simulink library "lib_finite_difference_filtered_derivative"  (R2023a)
settings: Solver=VariableStepAuto  StartTime=0.0  StopTime=10.0  RelTol=1e-3
undefined symbols (not defined in the file): bit
libraries: lib_conversion x4, lib_finite_difference_derivative x1, lib_iir_filter x1
settings Model: Creator=RAN2OFO  LastModifiedBy=xiaoqiang.yuan
settings OptimizationCC: ReuseModelBlockBuffer=off

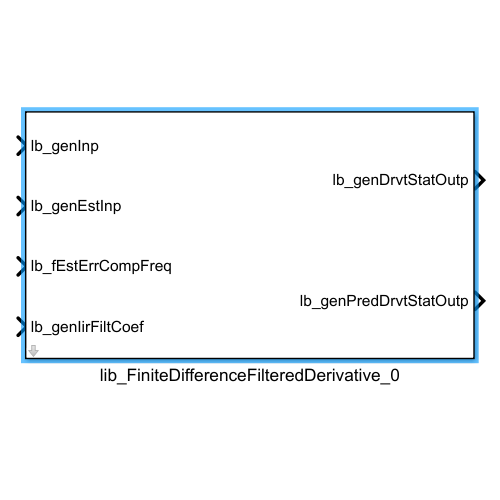
[thumbnail: Simulink's stored preview of the top-level diagram]
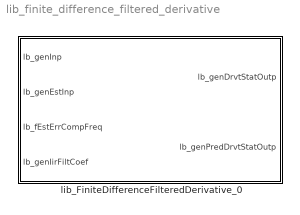
== system lib_finite_difference_filtered_derivative ==
  lib_FiniteDifferenceFilteredDerivative_0 : Subsystem  mask{lb_parSampTime=0.0005, lb_parInpMaxVal=100, lb_parInpEstErrMaxVal=0.1, lb_parInpDiffMaxVal=0.1, lb_parMaxEstErrCompFreq=4000, lb_parFltrCoefMaxVal=0.7, lb_genOutpUpLim=5000, lb_genOutpLowLim=-5000, lb_parOutpPekPhy=4096, lb_parAngInpMode=on, lb_parOutpDataType=fixdt(1,16,2^-3,0)}
      mask prompts: lb_parSampTime "Sampling time [s]:"; lb_parInpMaxVal "Maximum input [iu]:"; lb_parInpEstErrMaxVal "Maximum input estimation error [iu]:"; lb_parInpDiffMaxVal "Maximum input variation [iu]:"; lb_parMaxEstErrCompFreq "Maximum estimation error compensation frequency [Hz]:"; lb_parFltrCoefMaxVal "IIR filter coefficient max value:"; lb_genOutpUpLim "First state output upper limit [ou]:"; lb_genOutpLowLim "First state output lower limit [ou]:"; lb_parOutpPekPhy "Peak output physical value:"; lb_parAngInpMode "Angle input mode"; lb_parOutpDataType "Output data type:"
      mask init:
      | inpEstErrMaxVal = double(lb_parInpEstErrMaxVal);
      | inpMaxVal = double(lb_parInpMaxVal);
      | 
      | inpEstErrDataType = fi(2*inpMaxVal,1,32);
      | 
      | %% Req. XXX_ - Define data type for input variation
      | lb_parInpVrntDataType = Simulink.NumericType;
      | lb_parInpVrntDataType.DataTypeMode = 'Fixed-point: slope and bias scaling';
      | lb_parInpVrntDataType.Signedness = 'Signed';
      | lb_parInpVrntDataType.WordLength = 32;
      | switch lb_parAngInpMode
      |     case true
      |         lb_parInpVrntDataType.Slope = pi*2^-31;
      |     case false
      |         lb_parInpVrntDataType.Slope = 2^-(inpEstErrDataType.FractionLength);
      |  end
      | 
      | %% Req. XXX_ Define data type for product (u-u_pre)*cf
      | lb_parOper1MaxVal = inpEstErrMaxVal*lb_parMaxEstErrCompFreq;
      | lb_parOper1DataType = Simulink.NumericType;
      | lb_parOper1DataType.DataTypeMode= 'Fixed-point: unspecified scaling';
      | lb_parOper1DataType.Signedness = 'Signed';
      | lb_parOper1DataType.WordLength = 32;
      | 
      | %% Manage diagnostics for input variation sum
      | %% Restore any suppressed diagnostics
      | Simulink.restoreDiagnostic(gcb);
      | if lb_parAngInpMode == true
      |         Simulink.suppressDiagnostic([gcb,'/Add'],...
      |             'SimulinkFixedPoint:util:Overflowoccurred');
      | end
      mask TypeOptions lb_parFltrCoefMaxVal: lib_IirFilter_1/lb_parFltrCoefMaxVal
      mask TypeOptions lb_parAngInpMode: lib_FiniteDifferenceDerivative_1/lb_parAngInpMode
      mask DialogControl DescGroupVar Prompt: WEIFU motor control library
      mask DialogControl DescTextVar Prompt: Finite difference filtered derivative
      mask DialogControl dataTypeGroup Prompt: Data type

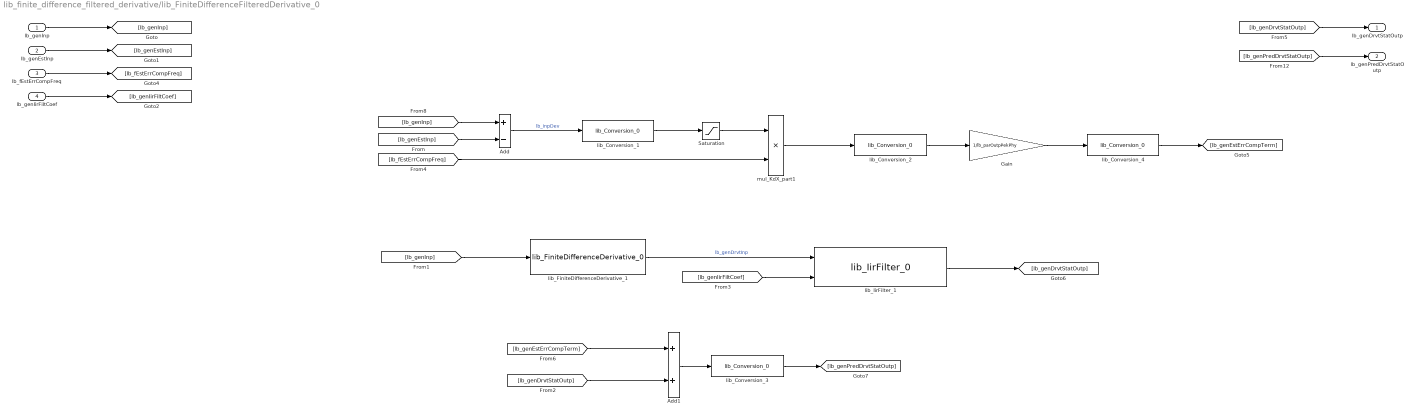
== system lib_finite_difference_filtered_derivative/lib_FiniteDifferenceFilteredDerivative_0 ==
  lb_genInp : Inport  PortDimensions=1
  lb_genEstInp : Inport  Port=2  PortDimensions=1
  lb_fEstErrCompFreq : Inport  Port=3
  lb_genIirFiltCoef : Inport  Port=4
  Add : Sum  Inputs=+-  OutDataTypeStr=Inherit: Inherit via back propagation  RndMeth=Simplest
  Add1 : Sum  OutDataTypeStr=Inherit: Inherit via back propagation  RndMeth=Simplest
  Gain : Gain  Gain=1/lb_parOutpPekPhy  OutDataTypeStr=Inherit: Inherit via back propagation
  Saturation : Saturate  UpperLimit=lb_parInpEstErrMaxVal  LowerLimit=-lb_parInpEstErrMaxVal
  lib_Conversion_1 : lib_conversion/lib_Conversion_0  lb_parDataType=lb_parInpVrntDataType  lb_parOutpMaxVal=[]  lb_parOutpMinVal=[]  lb_parSatFlag=off
  lib_Conversion_2 : lib_conversion/lib_Conversion_0  lb_parDataType=lb_parOper1DataType  lb_parOutpMaxVal=lb_parOper1MaxVal  lb_parOutpMinVal=[]  lb_parSatFlag=off
  lib_Conversion_3 : lib_conversion/lib_Conversion_0  lb_parDataType=lb_parOutpDataType  lb_parOutpMaxVal=[]  lb_parOutpMinVal=[]  lb_parSatFlag=off
  lib_Conversion_4 : lib_conversion/lib_Conversion_0  lb_parDataType=lb_parOutpDataType  lb_parOutpMaxVal=[]  lb_parOutpMinVal=[]  lb_parSatFlag=off
  lib_FiniteDifferenceDerivative_1 : lib_finite_difference_derivative/lib_FiniteDifferenceDerivative_0  lb_parSampTime=lb_parSampTime  lb_parMaxInpVar=lb_parInpDiffMaxVal  lb_parOutpPhyPek=lb_parOutpPekPhy  lb_parAngInpMode=on  lb_parOutpDataType=lb_parOutpDataType
      link override vss_AngleModeSelection: VariantControlMode=label  LabelModeActiveChoice=lb_parAngInpModeLbl
  lib_IirFilter_1 : lib_iir_filter/lib_IirFilter_0  lb_parMaxInpVal=lb_genOutpUpLim  lb_parFltrCoefMaxVal=lb_parFltrCoefMaxVal  lb_parBitNumMode=32-bit  lb_parOutpDataType=lb_parOutpDataType  lb_parFiltTypeMode=Low-pass
  mul_KdX_part1 : Product  OutDataTypeStr=Inherit: Inherit via back propagation  RndMeth=Simplest
  lb_genDrvtStatOutp : Outport  PortDimensions=1  VectorParamsAs1DForOutWhenUnconnected=off
  lb_genPredDrvtStatOutp : Outport  Port=2  PortDimensions=1  VectorParamsAs1DForOutWhenUnconnected=off
  wires:
  [lb_genIirFiltCoef] -> lib_IirFilter_1/2
  [lb_genDrvtStatOutp] -> Add1/2
  lib_IirFilter_1/1 -> [lb_genDrvtStatOutp]
  lib_FiniteDifferenceDerivative_1/1 -> lib_IirFilter_1/1  "lb_genDrvtInp"
  lb_genIirFiltCoef/1 -> [lb_genIirFiltCoef]
  [lb_genInp] -> lib_FiniteDifferenceDerivative_1/1
  [lb_genPredDrvtStatOutp] -> lb_genPredDrvtStatOutp/1
  [lb_genDrvtStatOutp] -> lb_genDrvtStatOutp/1
  mul_KdX_part1/1 -> lib_Conversion_2/1
  Add1/1 -> lib_Conversion_3/1
  [lb_fEstErrCompFreq] -> mul_KdX_part1/2
  [lb_genInp] -> Add/1
  [lb_genEstErrCompTerm] -> Add1/1
  lib_Conversion_2/1 -> Gain/1
  lb_genInp/1 -> [lb_genInp]
  [lb_genEstInp] -> Add/2
  lb_genEstInp/1 -> [lb_genEstInp]
  lib_Conversion_3/1 -> [lb_genPredDrvtStatOutp]
  lb_fEstErrCompFreq/1 -> [lb_fEstErrCompFreq]
  lib_Conversion_1/1 -> Saturation/1
  Add/1 -> lib_Conversion_1/1  "lb_inpDev"
  Saturation/1 -> mul_KdX_part1/1
  lib_Conversion_4/1 -> [lb_genEstErrCompTerm]
  Gain/1 -> lib_Conversion_4/1
